simulink model "control_EKF"  (R2024a)
settings: Solver=VariableStepAuto  StartTime=0.0  StopTime=4.5  RelTol=1e-3
values from neighbouring files (symbols this model uses):
  nlobj = nlmpc(nx, ny, 'MV', 1:nmv)    [init_mpc.m]    (also in init_mpc_EKF.m; init_mpc_constraint.m)
  params = [m1; m2; a1; a2; kj1; kj2; lbz-rj1; ac1; ac2]    [init_mpc.m]    (also in init_mpc_EKF.m; init_mpc_constraint.m; stateFcnRoboticArmEKF.m = uk(3:11))
  Ts_EKF = 0.001    [init_mpc_EKF.m]
libraries: sharedTrackingLibrary x1, mpclib x1, SignalEditorBlockLib x1
settings Model: Creator=berto  LastModifiedBy=berto

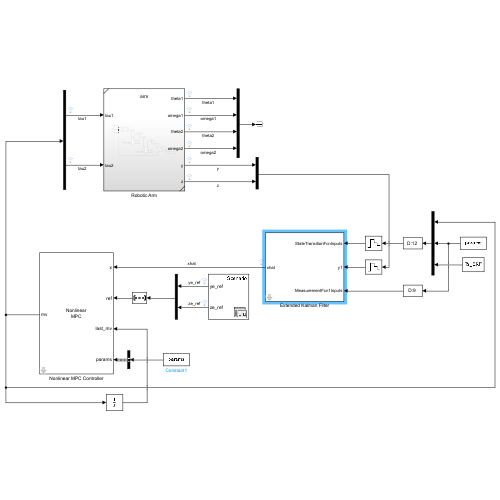
[thumbnail: Simulink's stored preview of the top-level diagram]
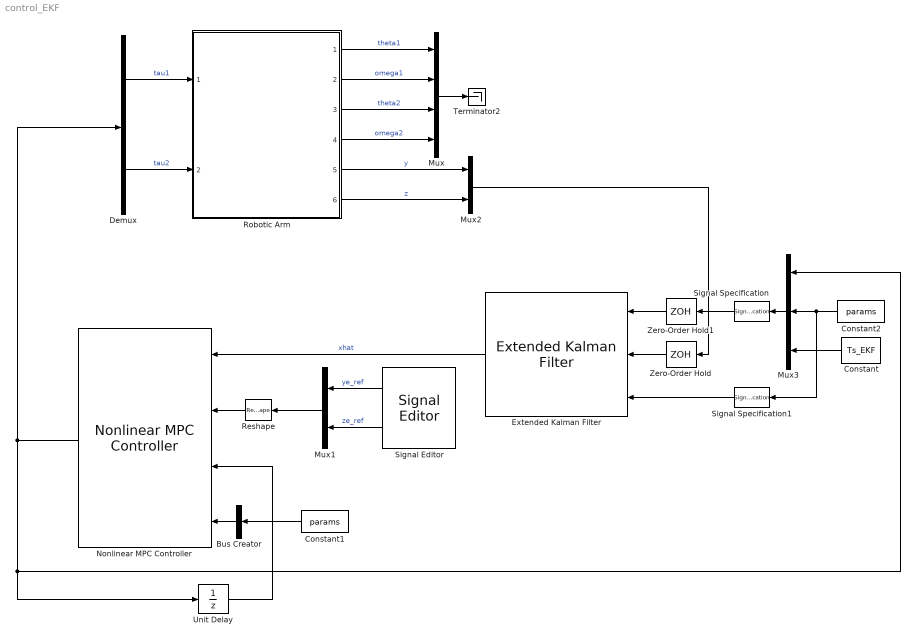
== system control_EKF ==
  Bus Creator : BusCreator  Inputs=1  OutDataTypeStr=Bus: paramsBusObject  NonVirtualBus=on
      settings: InheritFromInputs=off
  Constant : Constant  Value=Ts_EKF
  Constant1 : Constant  Value=params
  Constant2 : Constant  Value=params
  Demux : Demux  Outputs=2
  Extended Kalman Filter : sharedTrackingLibrary/Extended Kalman Filter  StateTransitionFcn=stateFcnRoboticArmEKF  HasStateTransitionJacobianFcn=off  HasAdditiveProcessNoise=Additive  ProcessNoise=QK  HasTimeVaryingProcessNoise=off  HasStateTransitionFcnExtraArgument=1  InitialState=x0  InitialStateCovariance=P0  MeasurementFcn1=outputFcnRoboticArmEKF  HasMeasurementJacobianFcn1=off  HasMeasurementEnablePort1=off  HasAdditiveMeasurementNoise1=Additive  MeasurementNoise1=RK  HasTimeVaryingMeasurementNoise1=off  HasMeasurementFcnExtraArgument1=1  HasMeasurementWrapping1=off  MeasurementFcn2=myMeasurementFcn  HasMeasurementJacobianFcn2=off  HasMeasurementEnablePort2=off  HasAdditiveMeasurementNoise2=Additive  MeasurementNoise2=1  HasTimeVaryingMeasurementNoise2=off  HasMeasurementFcnExtraArgument2=0  HasMeasurementWrapping2=off  MeasurementFcn3=myMeasurementFcn  HasMeasurementJacobianFcn3=off  HasMeasurementEnablePort3=off  HasAdditiveMeasurementNoise3=Additive  MeasurementNoise3=1  HasTimeVaryingMeasurementNoise3=off  HasMeasurementFcnExtraArgument3=0  HasMeasurementWrapping3=off  MeasurementFcn4=myMeasurementFcn  HasMeasurementJacobianFcn4=off  HasMeasurementEnablePort4=off  HasAdditiveMeasurementNoise4=Additive  MeasurementNoise4=1  HasTimeVaryingMeasurementNoise4=off  HasMeasurementFcnExtraArgument4=0  HasMeasurementWrapping4=off  MeasurementFcn5=myMeasurementFcn  HasMeasurementJacobianFcn5=off  HasMeasurementEnablePort5=off  HasAdditiveMeasurementNoise5=Additive  MeasurementNoise5=1  HasTimeVaryingMeasurementNoise5=off  HasMeasurementFcnExtraArgument5=0  HasMeasurementWrapping5=off  EnableMultirate=off  StateTransitionFcnSampleTime=1  MeasurementFcn1SampleTime=1  MeasurementFcn2SampleTime=1  MeasurementFcn3SampleTime=1  MeasurementFcn4SampleTime=1  MeasurementFcn5SampleTime=1  UseCurrentEstimator=on  OutputStateCovariance=off  DataType=double  SampleTime=Ts_EKF  NumberOfMeasurements=1
  Mux : Mux
  Mux1 : Mux  Inputs=2
  Mux2 : Mux  Inputs=2
  Mux3 : Mux  Inputs=3
  Nonlinear MPC Controller : mpclib/Nonlinear MPC Controller  nlmpcobj=nlobj  UseObjectTs=on  UseMEX=off  md_enabled=off  mvtarget_enabled=off  param_enabled=on  cost_enabled=off  mvseq_enabled=off  stateseq_enabled=off  ovseq_enabled=off  slack_enabled=off  status_enabled=off  ov_min=off  ov_max=off  mv_min=off  mv_max=off  mvrate_min=off  mvrate_max=off  state_min=off  state_max=off  ov_weight=off  mv_weight=off  mvrate_weight=off  ecr_weight=off  nlp_initialize=off
  Reshape : Reshape  OutputDimensionality=Row vector (2-D)
  Robotic Arm : Subsystem  ReferencedSubsystem=arm
  Signal Editor : SignalEditorBlockLib/Signal Editor  FileName=ref.mat  ActiveScenario=Scenario  ActiveSignal=ye_ref  IsBus=off  OutputBusObjectStr=Bus: BusObject  SampleTime=0  Interpolate=off  ZeroCross=off  OutputAfterFinalValue=Setting to zero  Unit=inherit  PreserveSignalName=on  ApplySigPropsToAllScenarios=on  ApplySigPropsToAllSignals=off
  Signal Specification : SignalSpecification  Dimensions=12
  Signal Specification1 : SignalSpecification  Dimensions=9
  Terminator2 : Terminator
  Unit Delay : UnitDelay  SampleTime=nlobj.Ts  HasFrameUpgradeWarning=on
  Zero-Order Hold : ZeroOrderHold  SampleTime=Ts_EKF
  Zero-Order Hold1 : ZeroOrderHold  SampleTime=Ts_EKF
  wires:
  Robotic Arm/1 -> Mux/1  "theta1"
  Robotic Arm/3 -> Mux/3  "theta2"
  Robotic Arm/2 -> Mux/2  "omega1"
  Robotic Arm/4 -> Mux/4  "omega2"
  Nonlinear MPC Controller/1 -> Unit Delay/1, Mux3/1, Demux/1
  Unit Delay/1 -> Nonlinear MPC Controller/3
  Demux/1 -> Robotic Arm/1  "tau1"
  Demux/2 -> Robotic Arm/2  "tau2"
  Constant1/1 -> Bus Creator/1
  Bus Creator/1 -> Nonlinear MPC Controller/4
  Reshape/1 -> Nonlinear MPC Controller/2
  Robotic Arm/5 -> Mux2/1  "y"
  Robotic Arm/6 -> Mux2/2  "z"
  Signal Editor/1 -> Mux1/1  "ye_ref"
  Signal Editor/2 -> Mux1/2  "ze_ref"
  Mux1/1 -> Reshape/1
  Mux/1 -> Terminator2/1
  Mux2/1 -> Zero-Order Hold/1
  Extended Kalman Filter/1 -> Nonlinear MPC Controller/1  "xhat"
  Mux3/1 -> Signal Specification/1
  Constant/1 -> Mux3/3
  Signal Specification/1 -> Zero-Order Hold1/1
  Zero-Order Hold/1 -> Extended Kalman Filter/2
  Zero-Order Hold1/1 -> Extended Kalman Filter/1
  Constant2/1 -> Signal Specification1/1, Mux3/2
  Signal Specification1/1 -> Extended Kalman Filter/3
